simulink model "PowE_lab4_controlledfullwaveRect"  (R2021b)
settings: Solver=VariableStepAuto  StartTime=0.0  StopTime=0.1  RelTol=1e-3
libraries: spsDetailedThyristorLib x4, spsVoltageMeasurementLib x3, spsACVoltageSourceLib x1, spsCurrentMeasurementLib x1, spsDCVoltageSourceLib x1, spsMeanLib x1, spsRMSLib x1, spsSeriesRLCBranchLib x1, spspowerguiLib x1
settings Model: Creator=kumaraditya  LastModifiedBy=Asus

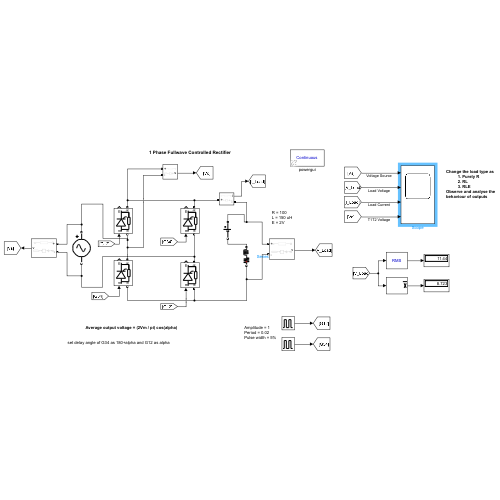
[thumbnail: Simulink's stored preview of the top-level diagram]
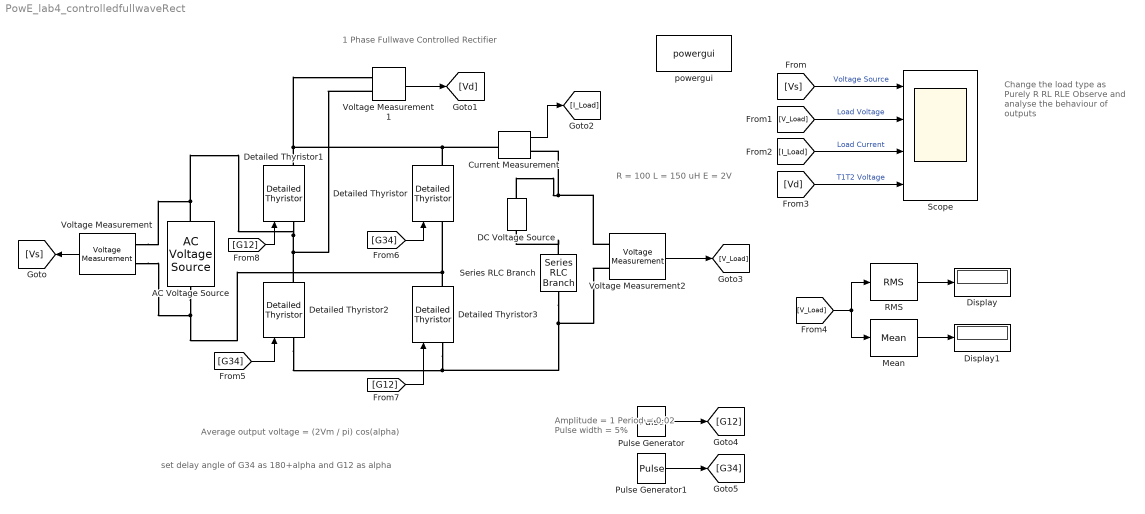
== system PowE_lab4_controlledfullwaveRect ==
  note: set delay angle of G34 as 180+alpha and G12 as alpha
  note: 1 Phase Fullwave Controlled Rectifier
  note: Average output voltage = (2Vm / pi) cos(alpha)
  note: Amplitude = 1
      | Period = 0.02
      | Pulse width = 5%
  note: R = 100
      | L = 150 uH
      | E = 2V
  note: Change the load type as
      | Purely R
      | RL
      | RLE
      | Observe and analyse the
      | behaviour of outputs
  AC Voltage Source : spsACVoltageSourceLib/AC Voltage Source  Amplitude=34  Phase=0  Frequency=50  SampleTime=0  Measurements=None  BusType=swing  Pref=10e3  Qref=0  Qmin=-inf  Qmax=+inf
  Current Measurement : spsCurrentMeasurementLib/Current Measurement  PhasorSimulation=off  OutputType=Complex  PSBequivalent=0
  DC Voltage Source : spsDCVoltageSourceLib/DC Voltage Source  Amplitude=5  Measurements=None
  Detailed Thyristor{,1..3} (4 alike) : spsDetailedThyristorLib/Detailed Thyristor  Ron=0.001  Lon=1e-3  Vf=0.8  IL=0.1  Tq=100e-6  IC=0  Rs=500  Cs=250e-9  Measurements=on
      settings: SourceProductBaseCode=PS
  Display : Display
  Display1 : Display
  Mean : spsMeanLib/Mean  Freq=60  Vinit=0  Ts=0
  Pulse Generator : DiscretePulseGenerator  PulseType=Time based  Period=0.02  PulseWidth=5  PhaseDelay=120*0.02/360
  Pulse Generator1 : DiscretePulseGenerator  PulseType=Time based  Period=0.02  PulseWidth=5  PhaseDelay=300*0.02/360
  RMS : spsRMSLib/RMS  TrueRMS=on  Freq=60  RMSInit=120  Ts=0
  Scope : Scope  NumInputPorts=4
  Series RLC Branch : spsSeriesRLCBranchLib/Series RLC Branch  LConnTagsString=__new0  RConnTagsString=__new0  BranchType=RL  Resistance=100  Inductance=100e-3  SetiL0=off  InitialCurrent=0  Capacitance=1e-6  Setx0=off  InitialVoltage=0  Measurements=None
  Voltage Measurement : spsVoltageMeasurementLib/Voltage Measurement  PhasorSimulation=off  OutputType=Complex  PSBequivalent=0
  Voltage Measurement1 : spsVoltageMeasurementLib/Voltage Measurement  PhasorSimulation=off  OutputType=Complex  PSBequivalent=0
  Voltage Measurement2 : spsVoltageMeasurementLib/Voltage Measurement  PhasorSimulation=off  OutputType=Complex  PSBequivalent=0
  powergui : spspowerguiLib/powergui  Priority=1  SimulationMode=Continuous  SampleTime=50e-6  frequency=60  Iterations=50  frequencyindice=50  Pbase=100e6  ErrMax=1e-4  UnitsV=kV  UnitsW=MW  buscounter=0  FunctionMessages=off  echomessages=off  EnableUseOfTLC=off  CurrentSourceSwitches=off  DisableSnubberDevices=off  DisableRonSwitches=off  DisableVfSwitches=off  DisplayEquations=off  AutomaticDiscreteSolvers=off  SolverType=Tustin/Backward Euler (TBE)  Interpol=off  ExternalGateDelay=off  methode=off  Ts=100  x0status=blocks  SPID=on  SwTol=0  HookPort=off  NonlinearTolerance=1e-4  nMaxIteration=100  ContinueOnMaxIteration=off  RestoreLinks=warning  ResistiveCurrentMeasurement=off  Frange=[0:2:500]  Ylog=off  Xlog=on  ShowGrid=off  save=off  variable=ZData  structure=0  ZoomFFT=off  StartTime=0.0  cycles=1  DisplayStyle=1  fundamental=60  FreqAxis=off  MaxFrequency=1000  frequencyindicesteady=1  RmsSteady=1  display=off
  wires:
  Mean/1 -> Display1/1
  [V_Load] -> RMS/1, Mean/1
  Voltage Measurement/1 -> [Vs]
  Current Measurement/1 -> [I_Load]
  [I_Load] -> Scope/3  "Load Current"
  [V_Load] -> Scope/2  "Load Voltage"
  RMS/1 -> Display/1
  [Vs] -> Scope/1  "Voltage Source"
  Voltage Measurement1/1 -> [Vd]
  Voltage Measurement2/1 -> [V_Load]
  [Vd] -> Scope/4  "T1T2 Voltage"
  Pulse Generator/1 -> [G12]
  Pulse Generator1/1 -> [G34]
  [G34] -> Detailed Thyristor2/1
  [G12] -> Detailed Thyristor3/1
  [G34] -> Detailed Thyristor/1
  [G12] -> Detailed Thyristor1/1
  connections:
  Current Measurement/LConn1 -- Detailed Thyristor/RConn1 -- Detailed Thyristor1/RConn1 -- Voltage Measurement1/LConn1
  Voltage Measurement1/LConn2 -- Detailed Thyristor2/RConn1 -- Voltage Measurement/LConn1 -- AC Voltage Source/RConn1 -- Detailed Thyristor1/LConn1
  AC Voltage Source/LConn1 -- Voltage Measurement/LConn2 -- Detailed Thyristor3/RConn1 -- Detailed Thyristor/LConn1
  Voltage Measurement2/LConn1 -- DC Voltage Source/RConn1 -- Current Measurement/RConn1
  Series RLC Branch/LConn1 -- Voltage Measurement2/LConn2 -- Detailed Thyristor3/LConn1 -- Detailed Thyristor2/LConn1
  Series RLC Branch/RConn1 -- DC Voltage Source/LConn1
